simulink library "write_txt_file"  (Simulink 8.2)
settings: Solver=ode45  StartTime=0.0  StopTime=10.0  RelTol=1e-3
settings Model: Creator=lena.frank  LastModifiedBy=drhf

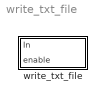
== system write_txt_file ==
  write_txt_file : Subsystem  mask{clear=off, filename='testout.txt'}
      mask prompts: clear "clear existing file"
      mask help:
      | This function writes the input data to a ascii-txt-file, so it can be opened with an usual editor.
      | The data is only written, when the enable signal is 1.
      | It's possible to append data to an existing file or to clear the file before writing.
      |
      | INPUT VECTOR
      |   in         : input data
      |   enable : signal [0,1]
      mask Help: web(fullfile(path_carnot('help'),'write_txt_file.html'),'-helpbrowser')

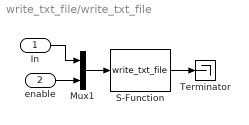
== system write_txt_file/write_txt_file ==
  In : Inport
  enable : Inport  Port=2
  Mux1 : Mux  Inputs=2
  S-Function : S-Function  FunctionName=write_txt_file  Parameters=clear filename  EnableBusSupport=off
  Terminator : Terminator
  wires:
  S-Function/1 -> Terminator/1
  Mux1/1 -> S-Function/1
  In/1 -> Mux1/1
  enable/1 -> Mux1/2
